simulink model "tram_with_battery"  (R2019b)
settings: Solver=VariableStepAuto  StartTime=0.0  StopTime=2360
values from neighbouring files (symbols this model uses):
  B = Tfriction/rated_speed_motor    (= 0.814101549937)    [Tram_battery.m]
  Cn = Np*Cn1    (= 153)    [Tram_battery.m]
  Cth = 240e3    (= 240000)    [Tram_battery.m]
  d = 680e-3    (= 0.68)    [Tram_battery.m]
  distance = [0,1,1.1,3,3.1,4,4.1,6,6.1,8,8.1,9,9.1,9.9,10]    [Tram_battery.m]
  E = Van-Ra*Ian    (= 540)    [Tram_battery.m]
  Gair = Kair*A_exchange    (= 100)    [Tram_battery.m]
  Gliquid = Kliquid*A_exchange    (= 1000)    [Tram_battery.m]
  Ien = 5    [Tram_battery.m]
  J_eq = m_full_load*((speed_tram/3.6)^2)/(rated_speed_motor^2)    (= 85.9801387874)    [Tram_battery.m]
  K = Tn/(Ian*Ien)    (= 1.06322065076)    [Tram_battery.m]
  kp_a = par_regi.Kp    [Tram_battery.m]
  kp_e = par_rege.Kp    [Tram_battery.m]
  kp_O = par_reg_speed.Kp    [Tram_battery.m]
  La = tau_a*Ra    (= 0.00385714285714)    [Tram_battery.m]
  Le = Re*tau_e    (= 1.2)    [Tram_battery.m]
  Ra = (1-efficiency)*Van/Ian    (= 0.385714285714)    [Tram_battery.m]
  rated_speed_motor = Or*(2*pi)/60    (= 101.578162466)    [Tram_battery.m]
  Re = Ven/Ien    (= 12)    [Tram_battery.m]
  rho = 13/74    (= 0.175675675676)    [Tram_battery.m]
  Rs1 = 3.6e-3    (= 0.0036)    [Tram_battery.m]
  SatLow_Va = -Van    (= -600)    [Tram_battery.m]
  SatLow_Ve = 0    [Tram_battery.m]
  SatUp_Va = Van    (= 600)    [Tram_battery.m]
  SatUp_Ve = Ven*1.1    (= 66)    [Tram_battery.m]
  Tfriction = Tn/10    (= 82.6949395034)    [Tram_battery.m]
  Ti_a = kp_a/ki_a    [Tram_battery.m]
  Ti_e = kp_e/ki_e    [Tram_battery.m]
  Ti_O = kp_O/ki_O    [Tram_battery.m]
  Tn = Pmec_eq/rated_speed_motor    (= 826.949395034)    [Tram_battery.m]
  Tslope = m_full_load*9.81*sin(theta)*d/2*rho    [Tram_battery.m]
undefined symbols (not defined in the file or in its folder): Q_init, Temperature_BP
libraries: simulink x2, drivingcycle_lib x1, powerlib x1
settings Model: Creator=secch  LastModifiedBy=secch
settings SolverCC: AlgebraicLoopSolver=LineSearch

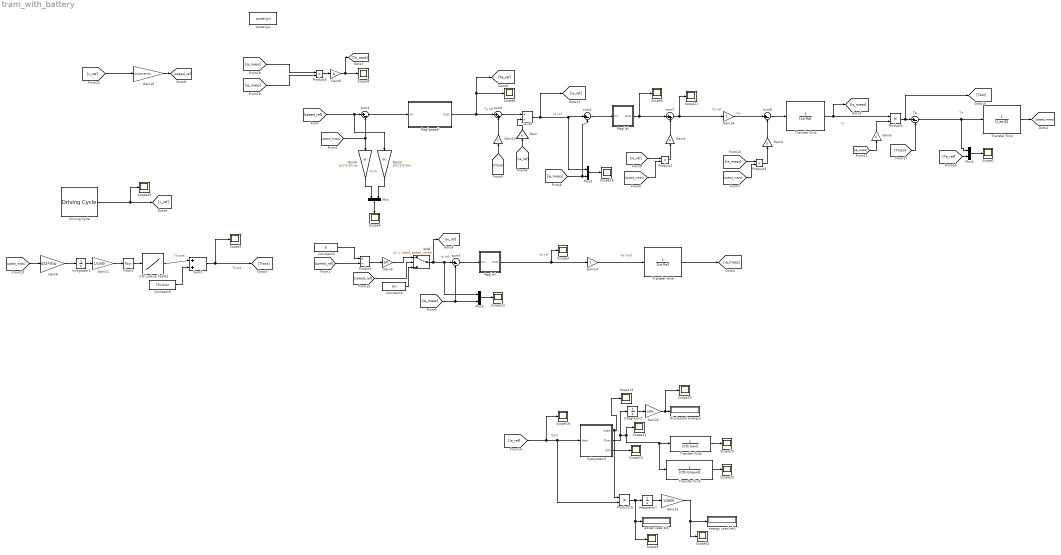
== system tram_with_battery ==
  note: km/h
  note: ia
  note: Va ref
  note: Ve load
  note: ie ref
  note: Te
  note: Ia ref
  note: Te ref
  note: Tload
  note: Tslope
  note: Ve ref
  note: Va
  note: Ibatt
  1-D Lookup Table1 : Lookup_n-D  NumberOfTableDimensions=1  BreakpointsForDimension1=distance  Table=Tslope  InternalRulePriority=Speed  RndMeth=Simplest  InputSameDT=on
  Constant3 : Constant  Value=E
  Constant4 : Constant  Value=Ien
  Constant9 : Constant  Value=Tfriction
  Dissipated energy2 : Display
  Driving Cycle : drivingcycle_lib/Driving Cycle  CycleName=NEDC  CycleRepeatsForever=off
      settings: SourceProductName=Driving Cycle Blockset
  Floor1 : Rounding
  Gain{,1,4..5,8} (5 alike) : Gain  Gain=K
  Gain10 : Gain
  Gain11 : Gain  Gain=1/1000
  Gain13 : Gain
  Gain14 : Gain
  Gain16 : Gain  Gain=1/(d/2*3.6*rho)
  Gain2 : Gain  Gain=d/2*3.6*rho
  Gain22 : Gain  Gain=1/3600
  Gain23 : Gain  Gain=1/3600
  Gain3 : Gain  Gain=1/K
  Gain6 : Gain  Gain=d/2*3.6*rho
  Gain9 : Gain  Gain=d/2*rho
  Integrator1 : Integrator
  Integrator2 : Integrator
  Integrator7 : Integrator
  Mux{,1..2,4} (4 alike) : Mux  Inputs=2
  Product : Product  Inputs=*/
  Product15 : Product  Inputs=**
  Product{2..5} (4 alike) : Product
  Reg(ia) : Subsystem
  Reg(ie) : Subsystem
  Reg(speed) : Subsystem
  Scope{1..6,8..13,16,18,21,23..24,29..30,51} (20 alike) : Scope
  Subsystem3 : Subsystem  mask{Em=|, R0=0.0036, SOC_BP=|, BattCap=31, SOC_ini=100, Ns=100, Np=3}
      mask Em=|
      | [3;
      | 3.5 ;
      | 3.67 ;
      | 3.7 ;
      | 3.71 ;
      | 3.72 ;
      | 3.73 ;
      | 3.74 ;
      | 3.75 ;
      | 3.84;
      | 4.2]
      mask SOC_BP=|
      | [0
      | 0.1
      | 0.2
      | 0.3
      | 0.4
      | 0.5
      | 0.6
      | 0.7
      | 0.8
      | 0.9
      | 1]
      mask prompts: Em "Open circuit voltage table data, Em [V]:"; R0 "Series resistance R0 [Ohm]:"; SOC_BP "State of charge breakpoints, SOC_BP []"; BattCap "Battery capacity, BattCap [Ah]"; SOC_ini "SOC ini [%]"; Ns "Num Series"; Np "Num Parallel"
      mask DialogControl Control3 Prompt: Single Module Data
      mask DialogControl Control2 Prompt: Connections
  Sum2 : Sum  Inputs=|++
  Te : Sum  Inputs=|+-
  Transfer Fcn2 : TransferFcn  Denominator=[J_eq B]
  Transfer Fcn3 : TransferFcn  Denominator=[La Ra]
  Transfer Fcn4 : TransferFcn  Denominator=[Cth Gair]
  Transfer Fcn5 : TransferFcn  Denominator=[Cth Gliquid]
  Transfer Fcn6 : TransferFcn  Denominator=[Le Re]
  energy used wh1 : Display
  ia ref : Product  Inputs=*/
  ieref : Switch  Criteria=u2 > Threshold  Threshold=rated_speed_motor
  power used W1 : Display
  powergui : powerlib/powergui  Priority=1  SimulationMode=Continuous  SampleTime=50e-6  frequency=60  Iterations=50  frequencyindice=0  Pbase=100e6  ErrMax=1e-4  UnitsV=kV  UnitsW=MW  buscounter=0  FunctionMessages=off  echomessages=off  EnableUseOfTLC=off  CurrentSourceSwitches=off  DisableSnubberDevices=off  DisableRonSwitches=off  DisableVfSwitches=off  DisplayEquations=off  AutomaticDiscreteSolvers=off  SolverType=Tustin/Backward Euler (TBE)  Interpol=off  ExternalGateDelay=off  methode=off  Ts=100  x0status=blocks  SPID=on  SwTol=0  HookPort=off  NonlinearTolerance=1e-4  nMaxIteration=100  ContinueOnMaxIteration=off  RestoreLinks=warning  ResistiveCurrentMeasurement=off  Frange=[0:2:500]  Ylog=off  Xlog=on  ShowGrid=off  save=off  variable=ZData  structure=0  ZoomFFT=off  StartTime=0.0  cycles=1  DisplayStyle=1  fundamental=60  FreqAxis=off  MaxFrequency=1000  frequencyindicesteady=1  RmsSteady=1  display=off
      settings: SourceProductName=Simscape Electrical
  sum{1,3,8..9} (4 alike) : Sum  Inputs=|+-
  sum6 : Sum  Inputs=|++
  sum7 : Sum  Inputs=|++
  wires:
  sum3/1 -> Reg(speed)/1(In1)
  [speed_ref] -> Gain2/1, sum3/1
  sum8/1 -> Transfer Fcn3/1
  Transfer Fcn3/1 -> Product4/1, [ia_meas]
  Constant3/1 -> Product/1
  Gain3/1 -> ieref/1
  Product/1 -> Gain3/1
  Constant4/1 -> ieref/3
  1-D Lookup Table1/1 -> Sum2/1
  Constant9/1 -> Sum2/2
  [speed_meas] -> sum3/2, Gain6/1
  Transfer Fcn2/1 -> [speed_meas]
  [ie_ref] -> Gain/1
  [ia_meas] -> Mux1/2, sum1/2
  Product3/1 -> Gain4/1
  [Tload] -> Gain10/1
  [ie_ref] -> Product2/1
  Product2/1 -> Gain1/1
  [speed_meas] -> Product2/2
  [speed_meas] -> Product3/2
  [ie_meas] -> Product3/1
  ieref/1 -> [ie_ref], Mux2/1, sum9/1
  [ie_meas] -> Mux2/2, sum9/2
  Gain13/1 -> Transfer Fcn6/1
  Transfer Fcn6/1 -> [ie_meas]
  sum7/1 -> Gain14/1, Scope11/1
  Gain14/1 -> sum8/1
  [ie_meas] -> Gain5/1
  Gain/1 -> ia ref/2
  Gain1/1 -> sum7/2
  Gain4/1 -> sum8/2
  Gain5/1 -> Product4/2
  Floor1/1 -> 1-D Lookup Table1/1
  Integrator1/1 -> Gain11/1
  [speed_meas] -> Gain9/1
  Gain9/1 -> Integrator1/1
  sum6/1 -> ia ref/1
  Mux/1 -> Scope4/1
  [speed_ref] -> Product/2
  Gain11/1 -> Floor1/1
  [speed_ref] -> ieref/2
  sum1/1 -> Reg(ia)/1(In1)
  sum9/1 -> Reg(ie)/1(In1)
  Gain2/1 -> Mux/1
  Gain6/1 -> Mux/2
  Reg(ia)/1(Out1) -> Scope5/1, sum7/1
  Reg(ie)/1(Out1) -> Gain13/1, Scope3/1
  Mux1/1 -> Scope18/1
  Mux2/1 -> Scope12/1
  Mux4/1 -> Scope1/1
  [Te_ref] -> Mux4/2
  Product4/1 -> [Tem], Te/1
  Te/1 -> Mux4/1, Transfer Fcn2/1
  [Tload] -> Te/2
  Gain8/1 -> [Te_weak], Scope8/1
  Product5/1 -> Gain8/1
  [ia_meas] -> Product5/1
  [ie_meas] -> Product5/2
  [v_ref] -> Gain16/1
  Gain16/1 -> [speed_ref]
  Driving Cycle/2 -> Scope29/1, [v_ref]
  Transfer Fcn5/1 -> Scope23/1
  Subsystem3/3(SOC) -> Scope24/1
  Gain22/1 -> Scope30/1, Dissipated energy2/1
  Integrator7/1 -> Gain23/1
  Transfer Fcn4/1 -> Scope10/1
  Subsystem3/2(Ploss) -> Integrator2/1, Scope21/1, Transfer Fcn5/1, Transfer Fcn4/1
  Gain23/1 -> Scope51/1, energy used wh1/1
  Integrator2/1 -> Gain22/1
  Subsystem3/1(Vbatt) -> Scope13/1, Product15/1
  Product15/1 -> Integrator7/1, Scope9/1, power used W1/1
  Reg(speed)/1(Out1) -> [Te_ref], Scope6/1, sum6/1
  ia ref/1 -> [ia_ref], sum1/1, Mux1/1
  Sum2/1 -> [Tload], Scope2/1
  Gain10/1 -> sum6/2
  [ia_ref] -> Scope16/1, Product15/2, Subsystem3/1(Ibatt)

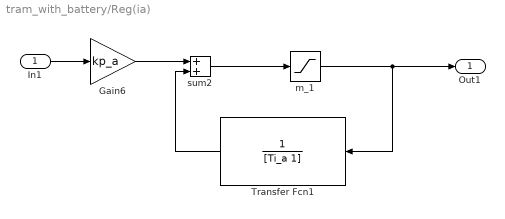
== system tram_with_battery/Reg(ia) ==
  In1 : Inport
  Gain6 : Gain  Gain=kp_a
  Transfer Fcn1 : TransferFcn  Denominator=[Ti_a 1]
  m_1 : Saturate  UpperLimit=SatUp_Va  LowerLimit=SatLow_Va
  sum2 : Sum
  Out1 : Outport
  wires:
  m_1/1 -> Out1/1, Transfer Fcn1/1
  In1/1 -> Gain6/1
  Transfer Fcn1/1 -> sum2/2
  Gain6/1 -> sum2/1
  sum2/1 -> m_1/1

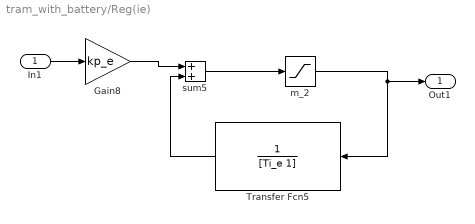
== system tram_with_battery/Reg(ie) ==
  In1 : Inport
  Gain8 : Gain  Gain=kp_e
  Transfer Fcn5 : TransferFcn  Denominator=[Ti_e 1]
  m_2 : Saturate  UpperLimit=SatUp_Ve  LowerLimit=SatLow_Ve
  sum5 : Sum
  Out1 : Outport
  wires:
  Transfer Fcn5/1 -> sum5/2
  In1/1 -> Gain8/1
  m_2/1 -> Out1/1, Transfer Fcn5/1
  Gain8/1 -> sum5/1
  sum5/1 -> m_2/1

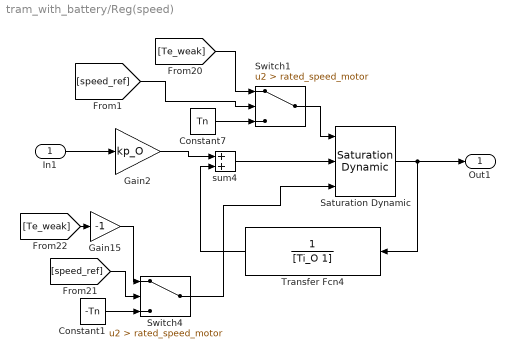
== system tram_with_battery/Reg(speed) ==
  In1 : Inport
  Constant1 : Constant  Value=-Tn
  Constant7 : Constant  Value=Tn
  Gain15 : Gain  Gain=-1
  Gain2 : Gain  Gain=kp_O
  Saturation Dynamic : simulink/Discontinuities/Saturation Dynamic  OutMin=[]  OutMax=[]  OutDataTypeStr=Inherit: Same as second input  OutDataType=fixdt(1, 16)  OutScaling=2^-10  DoSatur=off
  Switch1 : Switch  Criteria=u2 > Threshold  Threshold=rated_speed_motor
  Switch4 : Switch  Criteria=u2 > Threshold  Threshold=rated_speed_motor
  Transfer Fcn4 : TransferFcn  Denominator=[Ti_O 1]
  sum4 : Sum
  Out1 : Outport
  wires:
  Transfer Fcn4/1 -> sum4/2
  Switch4/1 -> Saturation Dynamic/3
  Saturation Dynamic/1 -> Out1/1, Transfer Fcn4/1
  Constant7/1 -> Switch1/3
  Switch1/1 -> Saturation Dynamic/1
  [Te_weak] -> Switch1/1
  In1/1 -> Gain2/1
  sum4/1 -> Saturation Dynamic/2
  [speed_ref] -> Switch1/2
  Gain2/1 -> sum4/1
  [speed_ref] -> Switch4/2
  Constant1/1 -> Switch4/3
  [Te_weak] -> Gain15/1
  Gain15/1 -> Switch4/1

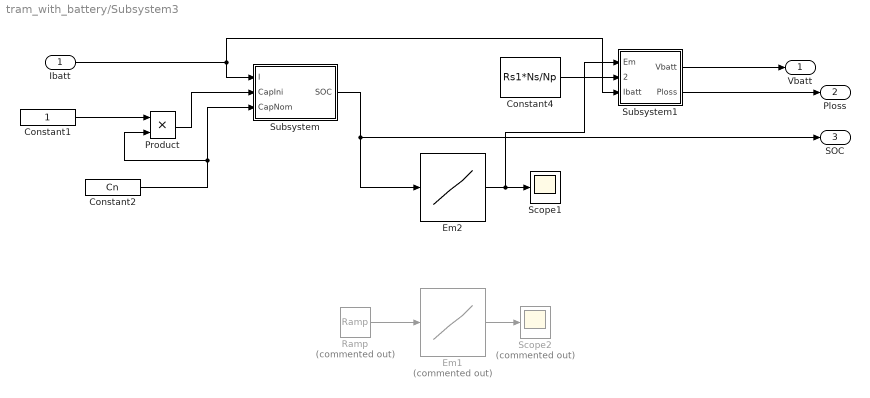
== system tram_with_battery/Subsystem3 ==
  Ibatt : Inport
  Constant1 : Constant  SampleTime=-1
  Constant2 : Constant  Value=Cn  SampleTime=-1
  Constant4 : Constant  Value=Rs1*Ns/Np  SampleTime=-1
  Em1 : Lookup_n-D  Commented=on  NumberOfTableDimensions=1  LookupTableObject=''  BreakpointsForDimension1=SOC_BP  BreakpointsForDimension2=Temperature_BP  Table=Em  InterpMethod=Cubic spline  ExtrapMethod=Clip  UseLastTableValue=on  InternalRulePriority=Speed  RndMeth=Simplest  InputSameDT=on
  Em2 : Lookup_n-D  NumberOfTableDimensions=1  LookupTableObject=''  BreakpointsForDimension1=[0,0.1,0.2,0.3,0.4,0.5,0.6,0.7,0.8,0.9,1]  BreakpointsForDimension2=Temperature_BP  Table=[500,550,567,570,571,572,573,574,575,584,600]  InterpMethod=Cubic spline  ExtrapMethod=Clip  UseLastTableValue=on  InternalRulePriority=Speed  RndMeth=Simplest  InputSameDT=on
  Product : Product
  Ramp : simulink/Sources/Ramp  Commented=on  slope=-0.5  start=0  InitialOutput=1
  Scope1 : Scope
  Scope2 : Scope  Commented=on
  Subsystem : Subsystem
  Subsystem1 : Subsystem
  Vbatt : Outport
  Ploss : Outport  Port=2
  SOC : Outport  Port=3
  wires:
  Constant1/1 -> Product/1
  Constant2/1 -> Product/2, Subsystem/3(CapNom)
  Product/1 -> Subsystem/2(CapIni)
  Constant4/1 -> Subsystem1/2(Rseries)
  Ibatt/1 -> Subsystem1/3(Ibatt), Subsystem/1(I)
  Em2/1 -> Scope1/1, Subsystem1/1(Em)
  Subsystem1/1(Vbatt) -> Vbatt/1
  Subsystem/1(SOC) -> Em2/1, SOC/1
  Subsystem1/2(Ploss) -> Ploss/1
  Em1/1 -> Scope2/1
  Ramp/1 -> Em1/1

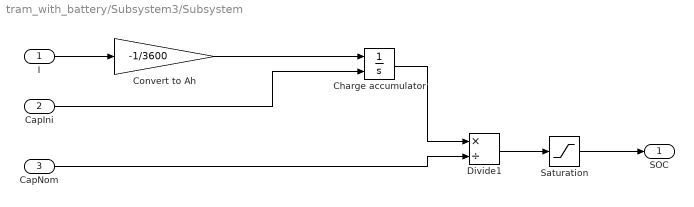
== system tram_with_battery/Subsystem3/Subsystem ==
  I : Inport
  CapIni : Inport  Port=2
  CapNom : Inport  Port=3
  Charge accumulator : Integrator  InitialConditionSource=external  InitialCondition=Q_init*3600  LowerSaturationLimit=0
  Convert to Ah : Gain  Gain=-1/3600
  Divide1 : Product  Inputs=*/
  Saturation : Saturate  UpperLimit=1  LowerLimit=0
  SOC : Outport
  wires:
  I/1 -> Convert to Ah/1
  Saturation/1 -> SOC/1
  Charge accumulator/1 -> Divide1/1
  CapNom/1 -> Divide1/2
  CapIni/1 -> Charge accumulator/2
  Convert to Ah/1 -> Charge accumulator/1
  Divide1/1 -> Saturation/1

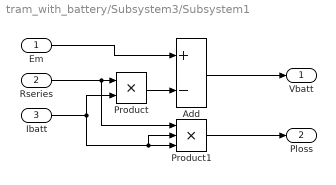
== system tram_with_battery/Subsystem3/Subsystem1 ==
  Em : Inport
  Rseries : Inport  Port=2
  Ibatt : Inport  Port=3
  Add : Sum  Inputs=+-
  Product : Product
  Product1 : Product  Inputs=3
  Vbatt : Outport
  Ploss : Outport  Port=2
  wires:
  Ibatt/1 -> Product/2, Product1/3, Product1/2
  Product1/1 -> Ploss/1
  Rseries/1 -> Product/1, Product1/1
  Em/1 -> Add/1
  Add/1 -> Vbatt/1
  Product/1 -> Add/2
